simulink model "main"  (R2023b)
settings: Solver=ode113  StartTime=tstart  StopTime=tend  RelTol=relTol  AbsTol=absTol
values from neighbouring files (symbols this model uses):
  D_init = JD_init - 2451545.0    (= 1484.5)    [EulerEquations.m]    (also in main_script.m)
  DCM_initial = targetDCM([26321453.5527815,	-132781955.130633,	-57571626.5531097]', R_princ)    [EulerEquations.m]    (also in main_script.m)
  EKF_P0 = eye(7)    [main_script.m]
  EKF_x0 = [0,0,0,0,0,0,0]    [main_script.m]
  inertia_p = [85.075, 0, 0; 0, 85.075, 0; 0, 0, 120.2515]    [omega_dot.m]
  omega_init = [0; 0; 0.01]    [EulerEquations.m]    (also in main_script.m = [0; 0; 0.0])
  state_ECI_init = [R_PQW_IJK*state_PQW_init(1:3)';R_PQW_IJK*state_PQW_init(4:6)']    [OrbitPropagation.m]
  theta = UT1_to_theta(UT1)    [EulerEquations.m]    (also in UT1_to_theta.m = rotz(-GMST*180/pi); main_script.m)
  tstart = 0    [EulerEquations.m]    (also in main_script.m)
  UT1 = [1,25,2004,00]    [EulerEquations.m]    (also in main_script.m)
undefined symbols (not defined in the file or in its folder): a_sun, e_sun, i_sun, M0_sun, n_sun, Om_sun, om_sun, R_princ
libraries: dspmathops x2, aerolibatmos2 x1, simulink x1, matrix_library x1
(part 2 of 2)

== matlab function main/Euler Equations/Euler Equations1 ==
  data: inertia_p input; M input; omegadot output; omega input
%% return omega_dot (zero torque)
function omegadot  = omega_dot(inertia_p, M, omega)
    %Euler eqns in principal axes
    omegadot = [ 1/inertia_p(1,1) * (M(1) - (inertia_p(3,3) - inertia_p(2,2)) * omega(2)*omega(3));
                 1/inertia_p(2,2) * (M(2) - (inertia_p(1,1) - inertia_p(3,3)) * omega(3)*omega(1));
                 1/inertia_p(3,3) * (M(3) - (inertia_p(2,2) - inertia_p(1,1)) * omega(1)*omega(2))];
end

== matlab function main/Quaternions/Initial Quaternions ==
  data: C input; quaternions_init output
%% Quaternions
function quaternions_init = inital_quaternions(C)
    beta_4sq = (0.25*(1+trace(C)));
    beta_1sq = (0.25*(1+2*C(1,1)- trace(C)));
    beta_2sq = (0.25*(1+2*C(2,2)- trace(C)));
    beta_3sq = (0.25*(1+2*C(3,3)- trace(C)));
    
    [maximum, max_ind] = max([beta_1sq, beta_2sq, beta_3sq, beta_4sq]);
    
    switch max_ind
        case 1
            beta_1 = sqrt(beta_1sq);
            beta_4 = (C(2,3) - C(3,2))/(4*beta_1);
            beta_3 = (C(3,1) + C(1,3))/(4*beta_1);
            beta_2 = (C(1,2) + C(2,1))/(4*beta_1);
        case 2
            beta_2 = sqrt(beta_2sq);
            beta_4 = (C(3,1) - C(1,3))/(4*beta_2);
            beta_3 = (C(2,3) + C(3,2))/(4*beta_2);
            beta_1 = (C(1,2) + C(2,1))/(4*beta_2);
        case 3
            beta_3 = sqrt(beta_3sq);
            beta_4 = (C(1,2) - C(2,1))/(4*beta_3);
            beta_2 = (C(2,3) + C(3,2))/(4*beta_3);
            beta_1 = (C(3,1) + C(1,3))/(4*beta_3);
           
        otherwise
            beta_4 = sqrt(beta_4sq);
            beta_3 = (C(1,2) - C(2,1))/(4*beta_4);
            beta_2 = (C(3,1) - C(1,3))/(4*beta_4);
            beta_1 = (C(2,3) - C(3,2))/(4*beta_4);   
    end
    
    quaternions_init = [beta_1; beta_2; beta_3; beta_4];
    quaternions_init =  quaternions_init/ norm(quaternions_init); %normalize
end

== matlab function main/Euler Angles/Euler Equations Euler ==
  data: omega input; euler input; eulerdot output
%% Kinematic Equation of motion for euler angles [phi, theta, psi]
function eulerdot = euler_dot(omega, euler)
     % phi_dot = (omega(1)* sin(euler(3)) + omega(2)*cos(euler(3)))/sin(euler(2));
     % theta_dot = omega(1) * cos(euler(3)) - omega(2) * sin(euler(3));
     % psi_dot = omega(3) - (omega(1)* sin(euler(3)) + omega(2)*cos(euler(3))) * cot(euler(2));
     % eulerdot = [phi_dot, theta_dot, psi_dot];
     phi = euler(1);
     theta = euler(2);
     psi = euler(3);

     eulerdot = 1/sin(theta)*[-sin(phi)*cos(theta), -cos(phi)*cos(theta), sin(theta);
                            cos(phi)*sin(theta), -sin(phi)*sin(theta), 0;
                            sin(phi), cos(phi), 0] * omega;
end

== matlab function main/Euler Angles/Initial Euler Angles ==
  data: C input; euler_init output
%% Euler Angles
function  euler_init = inital_euler(C)
    phi = atan2(C(1,3), C(2,3));
    theta = acos(C(3,3));
    psi = atan2(C(3,1), -C(3,2));
    euler_init = [phi; theta; psi];
end

== matlab function main/Euler Angles/Principal -> Inertial (Euler) ==
  data: euler input; omega_inertial_euler output; omega input; inertia_p input; L_inertial_euler output; R output
%% Transform Omega in inertial frame using Euler Angles
function [omega_inertial_euler, L_inertial_euler, R ] = principal_to_inertial(euler, omega, inertia_p)
    phi = euler(1);
    theta = euler(2);
    psi = euler(3);
    
    Rz = @(x)[cos(x), sin(x), 0;
              -sin(x), cos(x), 0;
              0, 0, 1];
    Rx =  @(x)[1, 0, 0;
              0, cos(x), sin(x),;
              0, -sin(x), cos(x)];


    %R = Rz(euler(1))*Rx(euler(2))*Rz(euler(3));

    R = [cos(phi)*cos(psi) - sin(phi)*cos(theta)*sin(psi), cos(phi)*sin(psi)+sin(phi)*cos(theta)*cos(psi), sin(phi)*sin(theta);
        -sin(phi)*cos(psi) - cos(phi)*cos(theta)*sin(psi), -sin(phi)*sin(psi)+cos(phi)*cos(theta)*cos(psi), cos(phi)*sin(theta);
        sin(theta)*sin(psi), -sin(theta)*cos(psi), cos(theta)];
    
    omega_inertial_euler = R' * omega;
    %inertia_inertial = R * inertia_p * R';
    %L_inertial_euler = inertia_inertial * omega_inertial_euler;
    L_inertial_euler = R' * inertia_p * omega;
end

== matlab function main/Quaternions/Principal -> Inertial (Quat) ==
  data: quaternions input; omega_inertial_quat output; omega input; inertia_p input; L_inertial_quat output; R output
%% Transform Omega in inertial frame using Quaternions
function  [omega_inertial_quat, L_inertial_quat, R] = principal_to_inertial(quaternions, omega, inertia_p)
    q4 = quaternions(4);
    q1 = quaternions(1);
    q2 = quaternions(2);
    q3 = quaternions(3);
    % R = [q0^2+q1^2-q2^2-q3^2, 2*q1*q2 + 2*q0*q3, 2*q1*q3 - 2*q0*q2;
    %      2*q1*q2 - 2*q0*q3, q0^2 - q1^2+q2^2 - q3^2, 2*q2*q3 + 2*q0*q1;
    %      2*q1*q3 + 2*q0*q2, 2*q2*q3 - 2*q0*q1, q0^2-q1^2-q2^2 + q3^2];
    R = (q4^2 - norm(quaternions(1:3))^2) * eye(3,3) + 2*quaternions(1:3)*quaternions(1:3)' -2*q4*[0, -q3, q2; q3, 0, -q1; -q2, q1, 0];
    omega_inertial_quat = R' * omega;
    L_inertial_quat = R' * inertia_p * omega; %inertia_inertial * omega_inertial_quat;
end

== matlab function main/Orbit Propagation/Orbit Propagation1 ==
  data: statedot output; state input
%% return equations of motion
function statedot  = state_dot(state)
    mu = 398600.435436; %Earth centered orbit
    statedot = zeros(6, 1);
    statedot(1:3) = state(4:6);
    statedot(4:6) = -mu * state(1:3)/(norm(state(1:3))^3);
end
